simulink model "Simulator_3D"  (R2018a)
settings: Solver=ode4  StartTime=0.0  StopTime=80  FixedStep=T  RelTol=1e-3
values from neighbouring files (symbols this model uses):
  A_w = 1*1.5/2    (= 0.75)    [init_Simulator.m]
  A_w2 = 1*0.27/2    (= 0.135)    [init_Simulator.m]
  epsilon_w = 0    [init_Simulator.m]
  epsilon_w2 = pi    (= 3.14159265359)    [init_Simulator.m]
  k_w = omega_w^2/g    (= 0.123862835563)    [init_Simulator.m]
  k_w2 = omega_w2^2/g    (= 0.447144836384)    [init_Simulator.m]
  Lc_0 = 7    [init_Simulator.m]
  omega_w = 2*pi/T_w    (= 1.10231321179)    [init_Simulator.m]
  omega_w2 = 2*pi/T_w2    (= 2.09439510239)    [init_Simulator.m]
  T = 1/30    (= 0.0333333333333)    [init_Simulator.m]
  w_dir = 1    [init_Simulator.m]
  w_dir2 = 1    [init_Simulator.m]
  zu_bar = X0_b(2) + Lc_0*sin(alpha_bar_0)    [init_Simulator.m]
libraries: vrlib x132
(part 3 of 6)

== system Simulator_3D/Subsystem/5 static wave points6/Subsystem16 ==
  t : Inport
  x : Inport  Port=2
  Subsystem : Subsystem
  Subsystem1 : Subsystem
  Sum1 : Sum  Inputs=++|
  Sum2 : Sum  Inputs=++|
  zeta : Outport
  theta : Outport  Port=2
  wires:
  x/1 -> Subsystem/2(x), Subsystem1/2(x)
  t/1 -> Subsystem/1(t), Subsystem1/1(t)
  Subsystem/1(zeta(x,t)) -> Sum2/2
  Sum2/1 -> zeta/1
  Subsystem1/1(zeta(x,t)) -> Sum2/1
  Subsystem/2(theta) -> Sum1/2
  Subsystem1/2(theta) -> Sum1/1
  Sum1/1 -> theta/1

== system Simulator_3D/Subsystem/5 static wave points7/Subsystem12 ==
  t : Inport
  x : Inport  Port=2
  Subsystem : Subsystem
  Subsystem1 : Subsystem
  Sum1 : Sum  Inputs=++|
  Sum2 : Sum  Inputs=++|
  zeta : Outport
  theta : Outport  Port=2
  wires:
  x/1 -> Subsystem/2(x), Subsystem1/2(x)
  t/1 -> Subsystem/1(t), Subsystem1/1(t)
  Subsystem/1(zeta(x,t)) -> Sum2/2
  Sum2/1 -> zeta/1
  Subsystem1/1(zeta(x,t)) -> Sum2/1
  Subsystem/2(theta) -> Sum1/2
  Subsystem1/2(theta) -> Sum1/1
  Sum1/1 -> theta/1

== system Simulator_3D/Subsystem/5 static wave points7/Subsystem13 ==
  t : Inport
  x : Inport  Port=2
  Subsystem : Subsystem
  Subsystem1 : Subsystem
  Sum1 : Sum  Inputs=++|
  Sum2 : Sum  Inputs=++|
  zeta : Outport
  theta : Outport  Port=2
  wires:
  Sum1/1 -> theta/1
  Subsystem1/2(theta) -> Sum1/1
  Subsystem/2(theta) -> Sum1/2
  Subsystem1/1(zeta(x,t)) -> Sum2/1
  Sum2/1 -> zeta/1
  Subsystem/1(zeta(x,t)) -> Sum2/2
  t/1 -> Subsystem1/1(t), Subsystem/1(t)
  x/1 -> Subsystem1/2(x), Subsystem/2(x)

== system Simulator_3D/Subsystem/5 static wave points7/Subsystem14 ==
  t : Inport
  x : Inport  Port=2
  Subsystem : Subsystem
  Subsystem1 : Subsystem
  Sum1 : Sum  Inputs=++|
  Sum2 : Sum  Inputs=++|
  zeta : Outport
  theta : Outport  Port=2
  wires:
  x/1 -> Subsystem/2(x), Subsystem1/2(x)
  t/1 -> Subsystem/1(t), Subsystem1/1(t)
  Subsystem/1(zeta(x,t)) -> Sum2/2
  Sum2/1 -> zeta/1
  Subsystem1/1(zeta(x,t)) -> Sum2/1
  Subsystem/2(theta) -> Sum1/2
  Subsystem1/2(theta) -> Sum1/1
  Sum1/1 -> theta/1

== system Simulator_3D/Subsystem/5 static wave points7/Subsystem15 ==
  t : Inport
  x : Inport  Port=2
  Subsystem : Subsystem
  Subsystem1 : Subsystem
  Sum1 : Sum  Inputs=++|
  Sum2 : Sum  Inputs=++|
  zeta : Outport
  theta : Outport  Port=2
  wires:
  Sum1/1 -> theta/1
  Subsystem1/2(theta) -> Sum1/1
  Subsystem/2(theta) -> Sum1/2
  Subsystem1/1(zeta(x,t)) -> Sum2/1
  Sum2/1 -> zeta/1
  Subsystem/1(zeta(x,t)) -> Sum2/2
  t/1 -> Subsystem1/1(t), Subsystem/1(t)
  x/1 -> Subsystem1/2(x), Subsystem/2(x)

== system Simulator_3D/Subsystem/5 static wave points7/Subsystem16 ==
  t : Inport
  x : Inport  Port=2
  Subsystem : Subsystem
  Subsystem1 : Subsystem
  Sum1 : Sum  Inputs=++|
  Sum2 : Sum  Inputs=++|
  zeta : Outport
  theta : Outport  Port=2
  wires:
  x/1 -> Subsystem/2(x), Subsystem1/2(x)
  t/1 -> Subsystem/1(t), Subsystem1/1(t)
  Subsystem/1(zeta(x,t)) -> Sum2/2
  Sum2/1 -> zeta/1
  Subsystem1/1(zeta(x,t)) -> Sum2/1
  Subsystem/2(theta) -> Sum1/2
  Subsystem1/2(theta) -> Sum1/1
  Sum1/1 -> theta/1

== system Simulator_3D/Subsystem/5 static wave points7/crest1 ==
  t : Inport
  Constant : Constant  Value=epsilon_w
  Constant1 : Constant
  Constant2 : Constant  Value=-k_w
  Divide : Product  Inputs=*/
  Gain : Gain  Gain=omega_w
  Sum1 : Sum  Inputs=-+-
  Trigonometric Function2 : Trigonometry  Operator=asin
  direction : Gain  Gain=w_dir
  x crest : Outport
  wires:
  Gain/1 -> Sum1/1
  Constant/1 -> Sum1/3
  t/1 -> direction/1
  Constant2/1 -> Divide/2
  direction/1 -> Gain/1
  Constant1/1 -> Trigonometric Function2/1
  Trigonometric Function2/1 -> Sum1/2
  Sum1/1 -> Divide/1
  Divide/1 -> x crest/1

== system Simulator_3D/Subsystem/5 static wave points7/crest2 ==
  t : Inport
  Constant : Constant  Value=epsilon_w2
  Constant1 : Constant
  Constant2 : Constant  Value=-k_w2
  Divide : Product  Inputs=*/
  Gain : Gain  Gain=omega_w2
  Sum1 : Sum  Inputs=-+-
  Trigonometric Function2 : Trigonometry  Operator=asin
  direction : Gain  Gain=w_dir2
  x crest : Outport
  wires:
  Divide/1 -> x crest/1
  Sum1/1 -> Divide/1
  Trigonometric Function2/1 -> Sum1/2
  Constant1/1 -> Trigonometric Function2/1
  direction/1 -> Gain/1
  Constant2/1 -> Divide/2
  t/1 -> direction/1
  Constant/1 -> Sum1/3
  Gain/1 -> Sum1/1

== system Simulator_3D/Subsystem/followers/Subsystem1 ==
  t : Inport
  x : Inport  Port=2
  Subsystem : Subsystem
  Subsystem1 : Subsystem
  Sum1 : Sum  Inputs=++|
  Sum2 : Sum  Inputs=++|
  zeta : Outport
  theta : Outport  Port=2
  wires:
  Sum1/1 -> theta/1
  Subsystem1/2(theta) -> Sum1/1
  Subsystem/2(theta) -> Sum1/2
  Subsystem1/1(zeta(x,t)) -> Sum2/1
  Sum2/1 -> zeta/1
  Subsystem/1(zeta(x,t)) -> Sum2/2
  t/1 -> Subsystem1/1(t), Subsystem/1(t)
  x/1 -> Subsystem1/2(x), Subsystem/2(x)

== system Simulator_3D/Subsystem/followers/Subsystem2 ==
  t : Inport
  x : Inport  Port=2
  Subsystem : Subsystem
  Subsystem1 : Subsystem
  Sum1 : Sum  Inputs=++|
  Sum2 : Sum  Inputs=++|
  zeta : Outport
  theta : Outport  Port=2
  wires:
  x/1 -> Subsystem/2(x), Subsystem1/2(x)
  t/1 -> Subsystem/1(t), Subsystem1/1(t)
  Subsystem/1(zeta(x,t)) -> Sum2/2
  Sum2/1 -> zeta/1
  Subsystem1/1(zeta(x,t)) -> Sum2/1
  Subsystem/2(theta) -> Sum1/2
  Subsystem1/2(theta) -> Sum1/1
  Sum1/1 -> theta/1

== system Simulator_3D/Subsystem/followers/Subsystem3 ==
  t : Inport
  x : Inport  Port=2
  Subsystem : Subsystem
  Subsystem1 : Subsystem
  Sum1 : Sum  Inputs=++|
  Sum2 : Sum  Inputs=++|
  zeta : Outport
  theta : Outport  Port=2
  wires:
  x/1 -> Subsystem/2(x), Subsystem1/2(x)
  t/1 -> Subsystem/1(t), Subsystem1/1(t)
  Subsystem/1(zeta(x,t)) -> Sum2/2
  Sum2/1 -> zeta/1
  Subsystem1/1(zeta(x,t)) -> Sum2/1
  Subsystem/2(theta) -> Sum1/2
  Subsystem1/2(theta) -> Sum1/1
  Sum1/1 -> theta/1

== system Simulator_3D/Subsystem/followers/Subsystem4 ==
  t : Inport
  x : Inport  Port=2
  Subsystem : Subsystem
  Subsystem1 : Subsystem
  Sum1 : Sum  Inputs=++|
  Sum2 : Sum  Inputs=++|
  zeta : Outport
  theta : Outport  Port=2
  wires:
  Sum1/1 -> theta/1
  Subsystem1/2(theta) -> Sum1/1
  Subsystem/2(theta) -> Sum1/2
  Subsystem1/1(zeta(x,t)) -> Sum2/1
  Sum2/1 -> zeta/1
  Subsystem/1(zeta(x,t)) -> Sum2/2
  t/1 -> Subsystem1/1(t), Subsystem/1(t)
  x/1 -> Subsystem1/2(x), Subsystem/2(x)

== system Simulator_3D/Subsystem/followers/Subsystem5 ==
  t : Inport
  x : Inport  Port=2
  Subsystem : Subsystem
  Subsystem1 : Subsystem
  Sum1 : Sum  Inputs=++|
  Sum2 : Sum  Inputs=++|
  zeta : Outport
  theta : Outport  Port=2
  wires:
  x/1 -> Subsystem/2(x), Subsystem1/2(x)
  t/1 -> Subsystem/1(t), Subsystem1/1(t)
  Subsystem/1(zeta(x,t)) -> Sum2/2
  Sum2/1 -> zeta/1
  Subsystem1/1(zeta(x,t)) -> Sum2/1
  Subsystem/2(theta) -> Sum1/2
  Subsystem1/2(theta) -> Sum1/1
  Sum1/1 -> theta/1

== system Simulator_3D/Subsystem/followers/Subsystem6 ==
  t : Inport
  x : Inport  Port=2
  Subsystem : Subsystem
  Subsystem1 : Subsystem
  Sum1 : Sum  Inputs=++|
  Sum2 : Sum  Inputs=++|
  zeta : Outport
  theta : Outport  Port=2
  wires:
  Sum1/1 -> theta/1
  Subsystem1/2(theta) -> Sum1/1
  Subsystem/2(theta) -> Sum1/2
  Subsystem1/1(zeta(x,t)) -> Sum2/1
  Sum2/1 -> zeta/1
  Subsystem/1(zeta(x,t)) -> Sum2/2
  t/1 -> Subsystem1/1(t), Subsystem/1(t)
  x/1 -> Subsystem1/2(x), Subsystem/2(x)

== system Simulator_3D/Subsystem/followers/Subsystem7 ==
  t : Inport
  x : Inport  Port=2
  Subsystem : Subsystem
  Subsystem1 : Subsystem
  Sum1 : Sum  Inputs=++|
  Sum2 : Sum  Inputs=++|
  zeta : Outport
  theta : Outport  Port=2
  wires:
  x/1 -> Subsystem/2(x), Subsystem1/2(x)
  t/1 -> Subsystem/1(t), Subsystem1/1(t)
  Subsystem/1(zeta(x,t)) -> Sum2/2
  Sum2/1 -> zeta/1
  Subsystem1/1(zeta(x,t)) -> Sum2/1
  Subsystem/2(theta) -> Sum1/2
  Subsystem1/2(theta) -> Sum1/1
  Sum1/1 -> theta/1

== system Simulator_3D/Subsystem/followers/Subsystem8 ==
  t : Inport
  x : Inport  Port=2
  Subsystem : Subsystem
  Subsystem1 : Subsystem
  Sum1 : Sum  Inputs=++|
  Sum2 : Sum  Inputs=++|
  zeta : Outport
  theta : Outport  Port=2
  wires:
  Sum1/1 -> theta/1
  Subsystem1/2(theta) -> Sum1/1
  Subsystem/2(theta) -> Sum1/2
  Subsystem1/1(zeta(x,t)) -> Sum2/1
  Sum2/1 -> zeta/1
  Subsystem/1(zeta(x,t)) -> Sum2/2
  t/1 -> Subsystem1/1(t), Subsystem/1(t)
  x/1 -> Subsystem1/2(x), Subsystem/2(x)

== system Simulator_3D/Subsystem1/Subsystem1/Subsystem ==
  note: Aw.Sin
  t : Inport
  x : Inport  Port=2
  Constant : Constant  Value=epsilon_w
  Gain : Gain  Gain=omega_w
  Gain1 : Gain  Gain=k_w
  Gain2 : Gain  Gain=A_w
  Sum : Sum  Inputs=++-
  Trigonometric Function : Trigonometry
  direction : Gain  Gain=w_dir
  zeta(x,t) : Outport
  wires:
  Gain/1 -> Sum/2
  Gain2/1 -> zeta(x,t)/1  "zeta(x,t)"
  Constant/1 -> Sum/1
  t/1 -> direction/1
  Gain1/1 -> Sum/3
  Trigonometric Function/1 -> Gain2/1
  x/1 -> Gain1/1
  direction/1 -> Gain/1
  Sum/1 -> Trigonometric Function/1

== system Simulator_3D/Subsystem1/Subsystem1/Subsystem1 ==
  note: Aw.Sin
  t : Inport
  x : Inport  Port=2
  Constant : Constant  Value=epsilon_w2
  Gain : Gain  Gain=omega_w2
  Gain1 : Gain  Gain=k_w2
  Gain2 : Gain  Gain=A_w2
  Sum : Sum  Inputs=++-
  Trigonometric Function : Trigonometry
  direction : Gain  Gain=w_dir2
  zeta(x,t) : Outport
  wires:
  Sum/1 -> Trigonometric Function/1
  direction/1 -> Gain/1
  x/1 -> Gain1/1
  Trigonometric Function/1 -> Gain2/1
  Gain1/1 -> Sum/3
  t/1 -> direction/1
  Constant/1 -> Sum/1
  Gain2/1 -> zeta(x,t)/1  "zeta(x,t)"
  Gain/1 -> Sum/2

== system Simulator_3D/Subsystem1/Subsystem10/Subsystem ==
  note: Aw.Sin
  t : Inport
  x : Inport  Port=2
  Constant : Constant  Value=epsilon_w
  Gain : Gain  Gain=omega_w
  Gain1 : Gain  Gain=k_w
  Gain2 : Gain  Gain=A_w
  Sum : Sum  Inputs=++-
  Trigonometric Function : Trigonometry
  direction : Gain  Gain=w_dir
  zeta(x,t) : Outport
  wires:
  Sum/1 -> Trigonometric Function/1
  direction/1 -> Gain/1
  x/1 -> Gain1/1
  Trigonometric Function/1 -> Gain2/1
  Gain1/1 -> Sum/3
  t/1 -> direction/1
  Constant/1 -> Sum/1
  Gain2/1 -> zeta(x,t)/1  "zeta(x,t)"
  Gain/1 -> Sum/2

== system Simulator_3D/Subsystem1/Subsystem10/Subsystem1 ==
  note: Aw.Sin
  t : Inport
  x : Inport  Port=2
  Constant : Constant  Value=epsilon_w2
  Gain : Gain  Gain=omega_w2
  Gain1 : Gain  Gain=k_w2
  Gain2 : Gain  Gain=A_w2
  Sum : Sum  Inputs=++-
  Trigonometric Function : Trigonometry
  direction : Gain  Gain=w_dir2
  zeta(x,t) : Outport
  wires:
  Gain/1 -> Sum/2
  Gain2/1 -> zeta(x,t)/1  "zeta(x,t)"
  Constant/1 -> Sum/1
  t/1 -> direction/1
  Gain1/1 -> Sum/3
  Trigonometric Function/1 -> Gain2/1
  x/1 -> Gain1/1
  direction/1 -> Gain/1
  Sum/1 -> Trigonometric Function/1

== system Simulator_3D/Subsystem1/Subsystem11/Subsystem ==
  note: Aw.Sin
  t : Inport
  x : Inport  Port=2
  Constant : Constant  Value=epsilon_w
  Gain : Gain  Gain=omega_w
  Gain1 : Gain  Gain=k_w
  Gain2 : Gain  Gain=A_w
  Sum : Sum  Inputs=++-
  Trigonometric Function : Trigonometry
  direction : Gain  Gain=w_dir
  zeta(x,t) : Outport
  wires:
  Gain/1 -> Sum/2
  Gain2/1 -> zeta(x,t)/1  "zeta(x,t)"
  Constant/1 -> Sum/1
  t/1 -> direction/1
  Gain1/1 -> Sum/3
  Trigonometric Function/1 -> Gain2/1
  x/1 -> Gain1/1
  direction/1 -> Gain/1
  Sum/1 -> Trigonometric Function/1

== system Simulator_3D/Subsystem1/Subsystem11/Subsystem1 ==
  note: Aw.Sin
  t : Inport
  x : Inport  Port=2
  Constant : Constant  Value=epsilon_w2
  Gain : Gain  Gain=omega_w2
  Gain1 : Gain  Gain=k_w2
  Gain2 : Gain  Gain=A_w2
  Sum : Sum  Inputs=++-
  Trigonometric Function : Trigonometry
  direction : Gain  Gain=w_dir2
  zeta(x,t) : Outport
  wires:
  Sum/1 -> Trigonometric Function/1
  direction/1 -> Gain/1
  x/1 -> Gain1/1
  Trigonometric Function/1 -> Gain2/1
  Gain1/1 -> Sum/3
  t/1 -> direction/1
  Constant/1 -> Sum/1
  Gain2/1 -> zeta(x,t)/1  "zeta(x,t)"
  Gain/1 -> Sum/2

== system Simulator_3D/Subsystem1/Subsystem12/Subsystem ==
  note: Aw.Sin
  t : Inport
  x : Inport  Port=2
  Constant : Constant  Value=epsilon_w
  Gain : Gain  Gain=omega_w
  Gain1 : Gain  Gain=k_w
  Gain2 : Gain  Gain=A_w
  Sum : Sum  Inputs=++-
  Trigonometric Function : Trigonometry
  direction : Gain  Gain=w_dir
  zeta(x,t) : Outport
  wires:
  Sum/1 -> Trigonometric Function/1
  direction/1 -> Gain/1
  x/1 -> Gain1/1
  Trigonometric Function/1 -> Gain2/1
  Gain1/1 -> Sum/3
  t/1 -> direction/1
  Constant/1 -> Sum/1
  Gain2/1 -> zeta(x,t)/1  "zeta(x,t)"
  Gain/1 -> Sum/2

== system Simulator_3D/Subsystem1/Subsystem12/Subsystem1 ==
  note: Aw.Sin
  t : Inport
  x : Inport  Port=2
  Constant : Constant  Value=epsilon_w2
  Gain : Gain  Gain=omega_w2
  Gain1 : Gain  Gain=k_w2
  Gain2 : Gain  Gain=A_w2
  Sum : Sum  Inputs=++-
  Trigonometric Function : Trigonometry
  direction : Gain  Gain=w_dir2
  zeta(x,t) : Outport
  wires:
  Gain/1 -> Sum/2
  Gain2/1 -> zeta(x,t)/1  "zeta(x,t)"
  Constant/1 -> Sum/1
  t/1 -> direction/1
  Gain1/1 -> Sum/3
  Trigonometric Function/1 -> Gain2/1
  x/1 -> Gain1/1
  direction/1 -> Gain/1
  Sum/1 -> Trigonometric Function/1

== system Simulator_3D/Subsystem1/Subsystem13/Subsystem ==
  note: Aw.Sin
  t : Inport
  x : Inport  Port=2
  Constant : Constant  Value=epsilon_w
  Gain : Gain  Gain=omega_w
  Gain1 : Gain  Gain=k_w
  Gain2 : Gain  Gain=A_w
  Sum : Sum  Inputs=++-
  Trigonometric Function : Trigonometry
  direction : Gain  Gain=w_dir
  zeta(x,t) : Outport
  wires:
  Gain/1 -> Sum/2
  Gain2/1 -> zeta(x,t)/1  "zeta(x,t)"
  Constant/1 -> Sum/1
  t/1 -> direction/1
  Gain1/1 -> Sum/3
  Trigonometric Function/1 -> Gain2/1
  x/1 -> Gain1/1
  direction/1 -> Gain/1
  Sum/1 -> Trigonometric Function/1

== system Simulator_3D/Subsystem1/Subsystem13/Subsystem1 ==
  note: Aw.Sin
  t : Inport
  x : Inport  Port=2
  Constant : Constant  Value=epsilon_w2
  Gain : Gain  Gain=omega_w2
  Gain1 : Gain  Gain=k_w2
  Gain2 : Gain  Gain=A_w2
  Sum : Sum  Inputs=++-
  Trigonometric Function : Trigonometry
  direction : Gain  Gain=w_dir2
  zeta(x,t) : Outport
  wires:
  Sum/1 -> Trigonometric Function/1
  direction/1 -> Gain/1
  x/1 -> Gain1/1
  Trigonometric Function/1 -> Gain2/1
  Gain1/1 -> Sum/3
  t/1 -> direction/1
  Constant/1 -> Sum/1
  Gain2/1 -> zeta(x,t)/1  "zeta(x,t)"
  Gain/1 -> Sum/2

== system Simulator_3D/Subsystem1/Subsystem14/Subsystem ==
  note: Aw.Sin
  t : Inport
  x : Inport  Port=2
  Constant : Constant  Value=epsilon_w
  Gain : Gain  Gain=omega_w
  Gain1 : Gain  Gain=k_w
  Gain2 : Gain  Gain=A_w
  Sum : Sum  Inputs=++-
  Trigonometric Function : Trigonometry
  direction : Gain  Gain=w_dir
  zeta(x,t) : Outport
  wires:
  Sum/1 -> Trigonometric Function/1
  direction/1 -> Gain/1
  x/1 -> Gain1/1
  Trigonometric Function/1 -> Gain2/1
  Gain1/1 -> Sum/3
  t/1 -> direction/1
  Constant/1 -> Sum/1
  Gain2/1 -> zeta(x,t)/1  "zeta(x,t)"
  Gain/1 -> Sum/2

== system Simulator_3D/Subsystem1/Subsystem14/Subsystem1 ==
  note: Aw.Sin
  t : Inport
  x : Inport  Port=2
  Constant : Constant  Value=epsilon_w2
  Gain : Gain  Gain=omega_w2
  Gain1 : Gain  Gain=k_w2
  Gain2 : Gain  Gain=A_w2
  Sum : Sum  Inputs=++-
  Trigonometric Function : Trigonometry
  direction : Gain  Gain=w_dir2
  zeta(x,t) : Outport
  wires:
  Gain/1 -> Sum/2
  Gain2/1 -> zeta(x,t)/1  "zeta(x,t)"
  Constant/1 -> Sum/1
  t/1 -> direction/1
  Gain1/1 -> Sum/3
  Trigonometric Function/1 -> Gain2/1
  x/1 -> Gain1/1
  direction/1 -> Gain/1
  Sum/1 -> Trigonometric Function/1

== system Simulator_3D/Subsystem1/Subsystem15/Subsystem ==
  note: Aw.Sin
  t : Inport
  x : Inport  Port=2
  Constant : Constant  Value=epsilon_w
  Gain : Gain  Gain=omega_w
  Gain1 : Gain  Gain=k_w
  Gain2 : Gain  Gain=A_w
  Sum : Sum  Inputs=++-
  Trigonometric Function : Trigonometry
  direction : Gain  Gain=w_dir
  zeta(x,t) : Outport
  wires:
  Gain/1 -> Sum/2
  Gain2/1 -> zeta(x,t)/1  "zeta(x,t)"
  Constant/1 -> Sum/1
  t/1 -> direction/1
  Gain1/1 -> Sum/3
  Trigonometric Function/1 -> Gain2/1
  x/1 -> Gain1/1
  direction/1 -> Gain/1
  Sum/1 -> Trigonometric Function/1

== system Simulator_3D/Subsystem1/Subsystem15/Subsystem1 ==
  note: Aw.Sin
  t : Inport
  x : Inport  Port=2
  Constant : Constant  Value=epsilon_w2
  Gain : Gain  Gain=omega_w2
  Gain1 : Gain  Gain=k_w2
  Gain2 : Gain  Gain=A_w2
  Sum : Sum  Inputs=++-
  Trigonometric Function : Trigonometry
  direction : Gain  Gain=w_dir2
  zeta(x,t) : Outport
  wires:
  Sum/1 -> Trigonometric Function/1
  direction/1 -> Gain/1
  x/1 -> Gain1/1
  Trigonometric Function/1 -> Gain2/1
  Gain1/1 -> Sum/3
  t/1 -> direction/1
  Constant/1 -> Sum/1
  Gain2/1 -> zeta(x,t)/1  "zeta(x,t)"
  Gain/1 -> Sum/2

== system Simulator_3D/Subsystem1/Subsystem16/Subsystem ==
  note: Aw.Sin
  t : Inport
  x : Inport  Port=2
  Constant : Constant  Value=epsilon_w
  Gain : Gain  Gain=omega_w
  Gain1 : Gain  Gain=k_w
  Gain2 : Gain  Gain=A_w
  Sum : Sum  Inputs=++-
  Trigonometric Function : Trigonometry
  direction : Gain  Gain=w_dir
  zeta(x,t) : Outport
  wires:
  Sum/1 -> Trigonometric Function/1
  direction/1 -> Gain/1
  x/1 -> Gain1/1
  Trigonometric Function/1 -> Gain2/1
  Gain1/1 -> Sum/3
  t/1 -> direction/1
  Constant/1 -> Sum/1
  Gain2/1 -> zeta(x,t)/1  "zeta(x,t)"
  Gain/1 -> Sum/2

== system Simulator_3D/Subsystem1/Subsystem16/Subsystem1 ==
  note: Aw.Sin
  t : Inport
  x : Inport  Port=2
  Constant : Constant  Value=epsilon_w2
  Gain : Gain  Gain=omega_w2
  Gain1 : Gain  Gain=k_w2
  Gain2 : Gain  Gain=A_w2
  Sum : Sum  Inputs=++-
  Trigonometric Function : Trigonometry
  direction : Gain  Gain=w_dir2
  zeta(x,t) : Outport
  wires:
  Gain/1 -> Sum/2
  Gain2/1 -> zeta(x,t)/1  "zeta(x,t)"
  Constant/1 -> Sum/1
  t/1 -> direction/1
  Gain1/1 -> Sum/3
  Trigonometric Function/1 -> Gain2/1
  x/1 -> Gain1/1
  direction/1 -> Gain/1
  Sum/1 -> Trigonometric Function/1

== system Simulator_3D/Subsystem1/Subsystem2/Subsystem ==
  note: Aw.Sin
  t : Inport
  x : Inport  Port=2
  Constant : Constant  Value=epsilon_w
  Gain : Gain  Gain=omega_w
  Gain1 : Gain  Gain=k_w
  Gain2 : Gain  Gain=A_w
  Sum : Sum  Inputs=++-
  Trigonometric Function : Trigonometry
  direction : Gain  Gain=w_dir
  zeta(x,t) : Outport
  wires:
  Sum/1 -> Trigonometric Function/1
  direction/1 -> Gain/1
  x/1 -> Gain1/1
  Trigonometric Function/1 -> Gain2/1
  Gain1/1 -> Sum/3
  t/1 -> direction/1
  Constant/1 -> Sum/1
  Gain2/1 -> zeta(x,t)/1  "zeta(x,t)"
  Gain/1 -> Sum/2

== system Simulator_3D/Subsystem1/Subsystem2/Subsystem1 ==
  note: Aw.Sin
  t : Inport
  x : Inport  Port=2
  Constant : Constant  Value=epsilon_w2
  Gain : Gain  Gain=omega_w2
  Gain1 : Gain  Gain=k_w2
  Gain2 : Gain  Gain=A_w2
  Sum : Sum  Inputs=++-
  Trigonometric Function : Trigonometry
  direction : Gain  Gain=w_dir2
  zeta(x,t) : Outport
  wires:
  Gain/1 -> Sum/2
  Gain2/1 -> zeta(x,t)/1  "zeta(x,t)"
  Constant/1 -> Sum/1
  t/1 -> direction/1
  Gain1/1 -> Sum/3
  Trigonometric Function/1 -> Gain2/1
  x/1 -> Gain1/1
  direction/1 -> Gain/1
  Sum/1 -> Trigonometric Function/1

== system Simulator_3D/Subsystem1/Subsystem3/Subsystem ==
  note: Aw.Sin
  t : Inport
  x : Inport  Port=2
  Constant : Constant  Value=epsilon_w
  Gain : Gain  Gain=omega_w
  Gain1 : Gain  Gain=k_w
  Gain2 : Gain  Gain=A_w
  Sum : Sum  Inputs=++-
  Trigonometric Function : Trigonometry
  direction : Gain  Gain=w_dir
  zeta(x,t) : Outport
  wires:
  Gain/1 -> Sum/2
  Gain2/1 -> zeta(x,t)/1  "zeta(x,t)"
  Constant/1 -> Sum/1
  t/1 -> direction/1
  Gain1/1 -> Sum/3
  Trigonometric Function/1 -> Gain2/1
  x/1 -> Gain1/1
  direction/1 -> Gain/1
  Sum/1 -> Trigonometric Function/1

== system Simulator_3D/Subsystem1/Subsystem3/Subsystem1 ==
  note: Aw.Sin
  t : Inport
  x : Inport  Port=2
  Constant : Constant  Value=epsilon_w2
  Gain : Gain  Gain=omega_w2
  Gain1 : Gain  Gain=k_w2
  Gain2 : Gain  Gain=A_w2
  Sum : Sum  Inputs=++-
  Trigonometric Function : Trigonometry
  direction : Gain  Gain=w_dir2
  zeta(x,t) : Outport
  wires:
  Sum/1 -> Trigonometric Function/1
  direction/1 -> Gain/1
  x/1 -> Gain1/1
  Trigonometric Function/1 -> Gain2/1
  Gain1/1 -> Sum/3
  t/1 -> direction/1
  Constant/1 -> Sum/1
  Gain2/1 -> zeta(x,t)/1  "zeta(x,t)"
  Gain/1 -> Sum/2

== system Simulator_3D/Subsystem1/Subsystem4/Subsystem ==
  note: Aw.Sin
  t : Inport
  x : Inport  Port=2
  Constant : Constant  Value=epsilon_w
  Gain : Gain  Gain=omega_w
  Gain1 : Gain  Gain=k_w
  Gain2 : Gain  Gain=A_w
  Sum : Sum  Inputs=++-
  Trigonometric Function : Trigonometry
  direction : Gain  Gain=w_dir
  zeta(x,t) : Outport
  wires:
  Sum/1 -> Trigonometric Function/1
  direction/1 -> Gain/1
  x/1 -> Gain1/1
  Trigonometric Function/1 -> Gain2/1
  Gain1/1 -> Sum/3
  t/1 -> direction/1
  Constant/1 -> Sum/1
  Gain2/1 -> zeta(x,t)/1  "zeta(x,t)"
  Gain/1 -> Sum/2

== system Simulator_3D/Subsystem1/Subsystem4/Subsystem1 ==
  note: Aw.Sin
  t : Inport
  x : Inport  Port=2
  Constant : Constant  Value=epsilon_w2
  Gain : Gain  Gain=omega_w2
  Gain1 : Gain  Gain=k_w2
  Gain2 : Gain  Gain=A_w2
  Sum : Sum  Inputs=++-
  Trigonometric Function : Trigonometry
  direction : Gain  Gain=w_dir2
  zeta(x,t) : Outport
  wires:
  Gain/1 -> Sum/2
  Gain2/1 -> zeta(x,t)/1  "zeta(x,t)"
  Constant/1 -> Sum/1
  t/1 -> direction/1
  Gain1/1 -> Sum/3
  Trigonometric Function/1 -> Gain2/1
  x/1 -> Gain1/1
  direction/1 -> Gain/1
  Sum/1 -> Trigonometric Function/1

== system Simulator_3D/Subsystem1/Subsystem5/Subsystem ==
  note: Aw.Sin
  t : Inport
  x : Inport  Port=2
  Constant : Constant  Value=epsilon_w
  Gain : Gain  Gain=omega_w
  Gain1 : Gain  Gain=k_w
  Gain2 : Gain  Gain=A_w
  Sum : Sum  Inputs=++-
  Trigonometric Function : Trigonometry
  direction : Gain  Gain=w_dir
  zeta(x,t) : Outport
  wires:
  Gain/1 -> Sum/2
  Gain2/1 -> zeta(x,t)/1  "zeta(x,t)"
  Constant/1 -> Sum/1
  t/1 -> direction/1
  Gain1/1 -> Sum/3
  Trigonometric Function/1 -> Gain2/1
  x/1 -> Gain1/1
  direction/1 -> Gain/1
  Sum/1 -> Trigonometric Function/1

== system Simulator_3D/Subsystem1/Subsystem5/Subsystem1 ==
  note: Aw.Sin
  t : Inport
  x : Inport  Port=2
  Constant : Constant  Value=epsilon_w2
  Gain : Gain  Gain=omega_w2
  Gain1 : Gain  Gain=k_w2
  Gain2 : Gain  Gain=A_w2
  Sum : Sum  Inputs=++-
  Trigonometric Function : Trigonometry
  direction : Gain  Gain=w_dir2
  zeta(x,t) : Outport
  wires:
  Sum/1 -> Trigonometric Function/1
  direction/1 -> Gain/1
  x/1 -> Gain1/1
  Trigonometric Function/1 -> Gain2/1
  Gain1/1 -> Sum/3
  t/1 -> direction/1
  Constant/1 -> Sum/1
  Gain2/1 -> zeta(x,t)/1  "zeta(x,t)"
  Gain/1 -> Sum/2

== system Simulator_3D/Subsystem1/Subsystem6/Subsystem ==
  note: Aw.Sin
  t : Inport
  x : Inport  Port=2
  Constant : Constant  Value=epsilon_w
  Gain : Gain  Gain=omega_w
  Gain1 : Gain  Gain=k_w
  Gain2 : Gain  Gain=A_w
  Sum : Sum  Inputs=++-
  Trigonometric Function : Trigonometry
  direction : Gain  Gain=w_dir
  zeta(x,t) : Outport
  wires:
  Sum/1 -> Trigonometric Function/1
  direction/1 -> Gain/1
  x/1 -> Gain1/1
  Trigonometric Function/1 -> Gain2/1
  Gain1/1 -> Sum/3
  t/1 -> direction/1
  Constant/1 -> Sum/1
  Gain2/1 -> zeta(x,t)/1  "zeta(x,t)"
  Gain/1 -> Sum/2

== system Simulator_3D/Subsystem1/Subsystem6/Subsystem1 ==
  note: Aw.Sin
  t : Inport
  x : Inport  Port=2
  Constant : Constant  Value=epsilon_w2
  Gain : Gain  Gain=omega_w2
  Gain1 : Gain  Gain=k_w2
  Gain2 : Gain  Gain=A_w2
  Sum : Sum  Inputs=++-
  Trigonometric Function : Trigonometry
  direction : Gain  Gain=w_dir2
  zeta(x,t) : Outport
  wires:
  Gain/1 -> Sum/2
  Gain2/1 -> zeta(x,t)/1  "zeta(x,t)"
  Constant/1 -> Sum/1
  t/1 -> direction/1
  Gain1/1 -> Sum/3
  Trigonometric Function/1 -> Gain2/1
  x/1 -> Gain1/1
  direction/1 -> Gain/1
  Sum/1 -> Trigonometric Function/1

== system Simulator_3D/Subsystem1/Subsystem7/Subsystem ==
  note: Aw.Sin
  t : Inport
  x : Inport  Port=2
  Constant : Constant  Value=epsilon_w
  Gain : Gain  Gain=omega_w
  Gain1 : Gain  Gain=k_w
  Gain2 : Gain  Gain=A_w
  Sum : Sum  Inputs=++-
  Trigonometric Function : Trigonometry
  direction : Gain  Gain=w_dir
  zeta(x,t) : Outport
  wires:
  Gain/1 -> Sum/2
  Gain2/1 -> zeta(x,t)/1  "zeta(x,t)"
  Constant/1 -> Sum/1
  t/1 -> direction/1
  Gain1/1 -> Sum/3
  Trigonometric Function/1 -> Gain2/1
  x/1 -> Gain1/1
  direction/1 -> Gain/1
  Sum/1 -> Trigonometric Function/1

== system Simulator_3D/Subsystem1/Subsystem7/Subsystem1 ==
  note: Aw.Sin
  t : Inport
  x : Inport  Port=2
  Constant : Constant  Value=epsilon_w2
  Gain : Gain  Gain=omega_w2
  Gain1 : Gain  Gain=k_w2
  Gain2 : Gain  Gain=A_w2
  Sum : Sum  Inputs=++-
  Trigonometric Function : Trigonometry
  direction : Gain  Gain=w_dir2
  zeta(x,t) : Outport
  wires:
  Sum/1 -> Trigonometric Function/1
  direction/1 -> Gain/1
  x/1 -> Gain1/1
  Trigonometric Function/1 -> Gain2/1
  Gain1/1 -> Sum/3
  t/1 -> direction/1
  Constant/1 -> Sum/1
  Gain2/1 -> zeta(x,t)/1  "zeta(x,t)"
  Gain/1 -> Sum/2

== system Simulator_3D/Subsystem1/Subsystem8/Subsystem ==
  note: Aw.Sin
  t : Inport
  x : Inport  Port=2
  Constant : Constant  Value=epsilon_w
  Gain : Gain  Gain=omega_w
  Gain1 : Gain  Gain=k_w
  Gain2 : Gain  Gain=A_w
  Sum : Sum  Inputs=++-
  Trigonometric Function : Trigonometry
  direction : Gain  Gain=w_dir
  zeta(x,t) : Outport
  wires:
  Sum/1 -> Trigonometric Function/1
  direction/1 -> Gain/1
  x/1 -> Gain1/1
  Trigonometric Function/1 -> Gain2/1
  Gain1/1 -> Sum/3
  t/1 -> direction/1
  Constant/1 -> Sum/1
  Gain2/1 -> zeta(x,t)/1  "zeta(x,t)"
  Gain/1 -> Sum/2

== system Simulator_3D/Subsystem1/Subsystem8/Subsystem1 ==
  note: Aw.Sin
  t : Inport
  x : Inport  Port=2
  Constant : Constant  Value=epsilon_w2
  Gain : Gain  Gain=omega_w2
  Gain1 : Gain  Gain=k_w2
  Gain2 : Gain  Gain=A_w2
  Sum : Sum  Inputs=++-
  Trigonometric Function : Trigonometry
  direction : Gain  Gain=w_dir2
  zeta(x,t) : Outport
  wires:
  Gain/1 -> Sum/2
  Gain2/1 -> zeta(x,t)/1  "zeta(x,t)"
  Constant/1 -> Sum/1
  t/1 -> direction/1
  Gain1/1 -> Sum/3
  Trigonometric Function/1 -> Gain2/1
  x/1 -> Gain1/1
  direction/1 -> Gain/1
  Sum/1 -> Trigonometric Function/1

== system Simulator_3D/Subsystem1/Subsystem9/Subsystem ==
  note: Aw.Sin
  t : Inport
  x : Inport  Port=2
  Constant : Constant  Value=epsilon_w
  Gain : Gain  Gain=omega_w
  Gain1 : Gain  Gain=k_w
  Gain2 : Gain  Gain=A_w
  Sum : Sum  Inputs=++-
  Trigonometric Function : Trigonometry
  direction : Gain  Gain=w_dir
  zeta(x,t) : Outport
  wires:
  Gain/1 -> Sum/2
  Gain2/1 -> zeta(x,t)/1  "zeta(x,t)"
  Constant/1 -> Sum/1
  t/1 -> direction/1
  Gain1/1 -> Sum/3
  Trigonometric Function/1 -> Gain2/1
  x/1 -> Gain1/1
  direction/1 -> Gain/1
  Sum/1 -> Trigonometric Function/1

== system Simulator_3D/Subsystem1/Subsystem9/Subsystem1 ==
  note: Aw.Sin
  t : Inport
  x : Inport  Port=2
  Constant : Constant  Value=epsilon_w2
  Gain : Gain  Gain=omega_w2
  Gain1 : Gain  Gain=k_w2
  Gain2 : Gain  Gain=A_w2
  Sum : Sum  Inputs=++-
  Trigonometric Function : Trigonometry
  direction : Gain  Gain=w_dir2
  zeta(x,t) : Outport
  wires:
  Sum/1 -> Trigonometric Function/1
  direction/1 -> Gain/1
  x/1 -> Gain1/1
  Trigonometric Function/1 -> Gain2/1
  Gain1/1 -> Sum/3
  t/1 -> direction/1
  Constant/1 -> Sum/1
  Gain2/1 -> zeta(x,t)/1  "zeta(x,t)"
  Gain/1 -> Sum/2

== system Simulator_3D/Subsystem2/Subsystem1/Subsystem ==
  note: Aw.Sin
  t : Inport
  x : Inport  Port=2
  Constant : Constant  Value=epsilon_w
  Gain : Gain  Gain=omega_w
  Gain1 : Gain  Gain=k_w
  Gain2 : Gain  Gain=A_w
  Gain5 : Gain  Gain=A_w*k_w
  Sum : Sum  Inputs=++-
  Trigonometric Function1 : Trigonometry  Operator=sincos
  Trigonometric Function2 : Trigonometry  Operator=atan
  direction : Gain  Gain=w_dir
  zeta(x,t) : Outport
  theta : Outport  Port=2
  wires:
  Trigonometric Function2/1 -> theta/1
  Gain5/1 -> Trigonometric Function2/1
  Trigonometric Function1/2 -> Gain5/1
  Gain/1 -> Sum/2
  Gain2/1 -> zeta(x,t)/1  "zeta(x,t)"
  Constant/1 -> Sum/1
  t/1 -> direction/1
  Gain1/1 -> Sum/3
  Trigonometric Function1/1 -> Gain2/1
  x/1 -> Gain1/1
  direction/1 -> Gain/1
  Sum/1 -> Trigonometric Function1/1

== system Simulator_3D/Subsystem2/Subsystem1/Subsystem1 ==
  note: Aw.Sin
  t : Inport
  x : Inport  Port=2
  Constant : Constant  Value=epsilon_w2
  Gain : Gain  Gain=omega_w2
  Gain1 : Gain  Gain=k_w2
  Gain2 : Gain  Gain=A_w2
  Gain5 : Gain  Gain=A_w2*k_w2
  Sum : Sum  Inputs=++-
  Trigonometric Function : Trigonometry  Operator=sincos
  Trigonometric Function1 : Trigonometry  Operator=atan
  direction : Gain  Gain=w_dir2
  zeta(x,t) : Outport
  theta : Outport  Port=2
  wires:
  Trigonometric Function/2 -> Gain5/1
  Trigonometric Function1/1 -> theta/1
  Gain5/1 -> Trigonometric Function1/1
  Sum/1 -> Trigonometric Function/1
  direction/1 -> Gain/1
  x/1 -> Gain1/1
  Trigonometric Function/1 -> Gain2/1
  Gain1/1 -> Sum/3
  t/1 -> direction/1
  Constant/1 -> Sum/1
  Gain2/1 -> zeta(x,t)/1  "zeta(x,t)"
  Gain/1 -> Sum/2

== system Simulator_3D/Subsystem2/Subsystem10/Subsystem ==
  note: Aw.Sin
  t : Inport
  x : Inport  Port=2
  Constant : Constant  Value=epsilon_w
  Gain : Gain  Gain=omega_w
  Gain1 : Gain  Gain=k_w
  Gain2 : Gain  Gain=A_w
  Gain5 : Gain  Gain=A_w*k_w
  Sum : Sum  Inputs=++-
  Trigonometric Function1 : Trigonometry  Operator=sincos
  Trigonometric Function2 : Trigonometry  Operator=atan
  direction : Gain  Gain=w_dir
  zeta(x,t) : Outport
  theta : Outport  Port=2
  wires:
  Trigonometric Function2/1 -> theta/1
  Gain5/1 -> Trigonometric Function2/1
  Trigonometric Function1/2 -> Gain5/1
  Gain/1 -> Sum/2
  Gain2/1 -> zeta(x,t)/1  "zeta(x,t)"
  Constant/1 -> Sum/1
  t/1 -> direction/1
  Gain1/1 -> Sum/3
  Trigonometric Function1/1 -> Gain2/1
  x/1 -> Gain1/1
  direction/1 -> Gain/1
  Sum/1 -> Trigonometric Function1/1

== system Simulator_3D/Subsystem2/Subsystem10/Subsystem1 ==
  note: Aw.Sin
  t : Inport
  x : Inport  Port=2
  Constant : Constant  Value=epsilon_w2
  Gain : Gain  Gain=omega_w2
  Gain1 : Gain  Gain=k_w2
  Gain2 : Gain  Gain=A_w2
  Gain5 : Gain  Gain=A_w2*k_w2
  Sum : Sum  Inputs=++-
  Trigonometric Function : Trigonometry  Operator=sincos
  Trigonometric Function1 : Trigonometry  Operator=atan
  direction : Gain  Gain=w_dir2
  zeta(x,t) : Outport
  theta : Outport  Port=2
  wires:
  Trigonometric Function/2 -> Gain5/1
  Trigonometric Function1/1 -> theta/1
  Gain5/1 -> Trigonometric Function1/1
  Sum/1 -> Trigonometric Function/1
  direction/1 -> Gain/1
  x/1 -> Gain1/1
  Trigonometric Function/1 -> Gain2/1
  Gain1/1 -> Sum/3
  t/1 -> direction/1
  Constant/1 -> Sum/1
  Gain2/1 -> zeta(x,t)/1  "zeta(x,t)"
  Gain/1 -> Sum/2

== system Simulator_3D/Subsystem2/Subsystem11/Subsystem ==
  note: Aw.Sin
  t : Inport
  x : Inport  Port=2
  Constant : Constant  Value=epsilon_w
  Gain : Gain  Gain=omega_w
  Gain1 : Gain  Gain=k_w
  Gain2 : Gain  Gain=A_w
  Gain5 : Gain  Gain=A_w*k_w
  Sum : Sum  Inputs=++-
  Trigonometric Function1 : Trigonometry  Operator=sincos
  Trigonometric Function2 : Trigonometry  Operator=atan
  direction : Gain  Gain=w_dir
  zeta(x,t) : Outport
  theta : Outport  Port=2
  wires:
  Sum/1 -> Trigonometric Function1/1
  direction/1 -> Gain/1
  x/1 -> Gain1/1
  Trigonometric Function1/1 -> Gain2/1
  Gain1/1 -> Sum/3
  t/1 -> direction/1
  Constant/1 -> Sum/1
  Gain2/1 -> zeta(x,t)/1  "zeta(x,t)"
  Gain/1 -> Sum/2
  Trigonometric Function1/2 -> Gain5/1
  Gain5/1 -> Trigonometric Function2/1
  Trigonometric Function2/1 -> theta/1

== system Simulator_3D/Subsystem2/Subsystem11/Subsystem1 ==
  note: Aw.Sin
  t : Inport
  x : Inport  Port=2
  Constant : Constant  Value=epsilon_w2
  Gain : Gain  Gain=omega_w2
  Gain1 : Gain  Gain=k_w2
  Gain2 : Gain  Gain=A_w2
  Gain5 : Gain  Gain=A_w2*k_w2
  Sum : Sum  Inputs=++-
  Trigonometric Function : Trigonometry  Operator=sincos
  Trigonometric Function1 : Trigonometry  Operator=atan
  direction : Gain  Gain=w_dir2
  zeta(x,t) : Outport
  theta : Outport  Port=2
  wires:
  Gain/1 -> Sum/2
  Gain2/1 -> zeta(x,t)/1  "zeta(x,t)"
  Constant/1 -> Sum/1
  t/1 -> direction/1
  Gain1/1 -> Sum/3
  Trigonometric Function/1 -> Gain2/1
  x/1 -> Gain1/1
  direction/1 -> Gain/1
  Sum/1 -> Trigonometric Function/1
  Gain5/1 -> Trigonometric Function1/1
  Trigonometric Function1/1 -> theta/1
  Trigonometric Function/2 -> Gain5/1

== system Simulator_3D/Subsystem2/Subsystem12/Subsystem ==
  note: Aw.Sin
  t : Inport
  x : Inport  Port=2
  Constant : Constant  Value=epsilon_w
  Gain : Gain  Gain=omega_w
  Gain1 : Gain  Gain=k_w
  Gain2 : Gain  Gain=A_w
  Gain5 : Gain  Gain=A_w*k_w
  Sum : Sum  Inputs=++-
  Trigonometric Function1 : Trigonometry  Operator=sincos
  Trigonometric Function2 : Trigonometry  Operator=atan
  direction : Gain  Gain=w_dir
  zeta(x,t) : Outport
  theta : Outport  Port=2
  wires:
  Trigonometric Function2/1 -> theta/1
  Gain5/1 -> Trigonometric Function2/1
  Trigonometric Function1/2 -> Gain5/1
  Gain/1 -> Sum/2
  Gain2/1 -> zeta(x,t)/1  "zeta(x,t)"
  Constant/1 -> Sum/1
  t/1 -> direction/1
  Gain1/1 -> Sum/3
  Trigonometric Function1/1 -> Gain2/1
  x/1 -> Gain1/1
  direction/1 -> Gain/1
  Sum/1 -> Trigonometric Function1/1

== system Simulator_3D/Subsystem2/Subsystem12/Subsystem1 ==
  note: Aw.Sin
  t : Inport
  x : Inport  Port=2
  Constant : Constant  Value=epsilon_w2
  Gain : Gain  Gain=omega_w2
  Gain1 : Gain  Gain=k_w2
  Gain2 : Gain  Gain=A_w2
  Gain5 : Gain  Gain=A_w2*k_w2
  Sum : Sum  Inputs=++-
  Trigonometric Function : Trigonometry  Operator=sincos
  Trigonometric Function1 : Trigonometry  Operator=atan
  direction : Gain  Gain=w_dir2
  zeta(x,t) : Outport
  theta : Outport  Port=2
  wires:
  Trigonometric Function/2 -> Gain5/1
  Trigonometric Function1/1 -> theta/1
  Gain5/1 -> Trigonometric Function1/1
  Sum/1 -> Trigonometric Function/1
  direction/1 -> Gain/1
  x/1 -> Gain1/1
  Trigonometric Function/1 -> Gain2/1
  Gain1/1 -> Sum/3
  t/1 -> direction/1
  Constant/1 -> Sum/1
  Gain2/1 -> zeta(x,t)/1  "zeta(x,t)"
  Gain/1 -> Sum/2

== system Simulator_3D/Subsystem2/Subsystem13/Subsystem ==
  note: Aw.Sin
  t : Inport
  x : Inport  Port=2
  Constant : Constant  Value=epsilon_w
  Gain : Gain  Gain=omega_w
  Gain1 : Gain  Gain=k_w
  Gain2 : Gain  Gain=A_w
  Gain5 : Gain  Gain=A_w*k_w
  Sum : Sum  Inputs=++-
  Trigonometric Function1 : Trigonometry  Operator=sincos
  Trigonometric Function2 : Trigonometry  Operator=atan
  direction : Gain  Gain=w_dir
  zeta(x,t) : Outport
  theta : Outport  Port=2
  wires:
  Sum/1 -> Trigonometric Function1/1
  direction/1 -> Gain/1
  x/1 -> Gain1/1
  Trigonometric Function1/1 -> Gain2/1
  Gain1/1 -> Sum/3
  t/1 -> direction/1
  Constant/1 -> Sum/1
  Gain2/1 -> zeta(x,t)/1  "zeta(x,t)"
  Gain/1 -> Sum/2
  Trigonometric Function1/2 -> Gain5/1
  Gain5/1 -> Trigonometric Function2/1
  Trigonometric Function2/1 -> theta/1

== system Simulator_3D/Subsystem2/Subsystem13/Subsystem1 ==
  note: Aw.Sin
  t : Inport
  x : Inport  Port=2
  Constant : Constant  Value=epsilon_w2
  Gain : Gain  Gain=omega_w2
  Gain1 : Gain  Gain=k_w2
  Gain2 : Gain  Gain=A_w2
  Gain5 : Gain  Gain=A_w2*k_w2
  Sum : Sum  Inputs=++-
  Trigonometric Function : Trigonometry  Operator=sincos
  Trigonometric Function1 : Trigonometry  Operator=atan
  direction : Gain  Gain=w_dir2
  zeta(x,t) : Outport
  theta : Outport  Port=2
  wires:
  Gain/1 -> Sum/2
  Gain2/1 -> zeta(x,t)/1  "zeta(x,t)"
  Constant/1 -> Sum/1
  t/1 -> direction/1
  Gain1/1 -> Sum/3
  Trigonometric Function/1 -> Gain2/1
  x/1 -> Gain1/1
  direction/1 -> Gain/1
  Sum/1 -> Trigonometric Function/1
  Gain5/1 -> Trigonometric Function1/1
  Trigonometric Function1/1 -> theta/1
  Trigonometric Function/2 -> Gain5/1

== system Simulator_3D/Subsystem2/Subsystem14/Subsystem ==
  note: Aw.Sin
  t : Inport
  x : Inport  Port=2
  Constant : Constant  Value=epsilon_w
  Gain : Gain  Gain=omega_w
  Gain1 : Gain  Gain=k_w
  Gain2 : Gain  Gain=A_w
  Gain5 : Gain  Gain=A_w*k_w
  Sum : Sum  Inputs=++-
  Trigonometric Function1 : Trigonometry  Operator=sincos
  Trigonometric Function2 : Trigonometry  Operator=atan
  direction : Gain  Gain=w_dir
  zeta(x,t) : Outport
  theta : Outport  Port=2
  wires:
  Trigonometric Function2/1 -> theta/1
  Gain5/1 -> Trigonometric Function2/1
  Trigonometric Function1/2 -> Gain5/1
  Gain/1 -> Sum/2
  Gain2/1 -> zeta(x,t)/1  "zeta(x,t)"
  Constant/1 -> Sum/1
  t/1 -> direction/1
  Gain1/1 -> Sum/3
  Trigonometric Function1/1 -> Gain2/1
  x/1 -> Gain1/1
  direction/1 -> Gain/1
  Sum/1 -> Trigonometric Function1/1

== system Simulator_3D/Subsystem2/Subsystem14/Subsystem1 ==
  note: Aw.Sin
  t : Inport
  x : Inport  Port=2
  Constant : Constant  Value=epsilon_w2
  Gain : Gain  Gain=omega_w2
  Gain1 : Gain  Gain=k_w2
  Gain2 : Gain  Gain=A_w2
  Gain5 : Gain  Gain=A_w2*k_w2
  Sum : Sum  Inputs=++-
  Trigonometric Function : Trigonometry  Operator=sincos
  Trigonometric Function1 : Trigonometry  Operator=atan
  direction : Gain  Gain=w_dir2
  zeta(x,t) : Outport
  theta : Outport  Port=2
  wires:
  Trigonometric Function/2 -> Gain5/1
  Trigonometric Function1/1 -> theta/1
  Gain5/1 -> Trigonometric Function1/1
  Sum/1 -> Trigonometric Function/1
  direction/1 -> Gain/1
  x/1 -> Gain1/1
  Trigonometric Function/1 -> Gain2/1
  Gain1/1 -> Sum/3
  t/1 -> direction/1
  Constant/1 -> Sum/1
  Gain2/1 -> zeta(x,t)/1  "zeta(x,t)"
  Gain/1 -> Sum/2

== system Simulator_3D/Subsystem2/Subsystem15/Subsystem ==
  note: Aw.Sin
  t : Inport
  x : Inport  Port=2
  Constant : Constant  Value=epsilon_w
  Gain : Gain  Gain=omega_w
  Gain1 : Gain  Gain=k_w
  Gain2 : Gain  Gain=A_w
  Gain5 : Gain  Gain=A_w*k_w
  Sum : Sum  Inputs=++-
  Trigonometric Function1 : Trigonometry  Operator=sincos
  Trigonometric Function2 : Trigonometry  Operator=atan
  direction : Gain  Gain=w_dir
  zeta(x,t) : Outport
  theta : Outport  Port=2
  wires:
  Sum/1 -> Trigonometric Function1/1
  direction/1 -> Gain/1
  x/1 -> Gain1/1
  Trigonometric Function1/1 -> Gain2/1
  Gain1/1 -> Sum/3
  t/1 -> direction/1
  Constant/1 -> Sum/1
  Gain2/1 -> zeta(x,t)/1  "zeta(x,t)"
  Gain/1 -> Sum/2
  Trigonometric Function1/2 -> Gain5/1
  Gain5/1 -> Trigonometric Function2/1
  Trigonometric Function2/1 -> theta/1

== system Simulator_3D/Subsystem2/Subsystem15/Subsystem1 ==
  note: Aw.Sin
  t : Inport
  x : Inport  Port=2
  Constant : Constant  Value=epsilon_w2
  Gain : Gain  Gain=omega_w2
  Gain1 : Gain  Gain=k_w2
  Gain2 : Gain  Gain=A_w2
  Gain5 : Gain  Gain=A_w2*k_w2
  Sum : Sum  Inputs=++-
  Trigonometric Function : Trigonometry  Operator=sincos
  Trigonometric Function1 : Trigonometry  Operator=atan
  direction : Gain  Gain=w_dir2
  zeta(x,t) : Outport
  theta : Outport  Port=2
  wires:
  Gain/1 -> Sum/2
  Gain2/1 -> zeta(x,t)/1  "zeta(x,t)"
  Constant/1 -> Sum/1
  t/1 -> direction/1
  Gain1/1 -> Sum/3
  Trigonometric Function/1 -> Gain2/1
  x/1 -> Gain1/1
  direction/1 -> Gain/1
  Sum/1 -> Trigonometric Function/1
  Gain5/1 -> Trigonometric Function1/1
  Trigonometric Function1/1 -> theta/1
  Trigonometric Function/2 -> Gain5/1

== system Simulator_3D/Subsystem2/Subsystem16/Subsystem ==
  note: Aw.Sin
  t : Inport
  x : Inport  Port=2
  Constant : Constant  Value=epsilon_w
  Gain : Gain  Gain=omega_w
  Gain1 : Gain  Gain=k_w
  Gain2 : Gain  Gain=A_w
  Gain5 : Gain  Gain=A_w*k_w
  Sum : Sum  Inputs=++-
  Trigonometric Function1 : Trigonometry  Operator=sincos
  Trigonometric Function2 : Trigonometry  Operator=atan
  direction : Gain  Gain=w_dir
  zeta(x,t) : Outport
  theta : Outport  Port=2
  wires:
  Trigonometric Function2/1 -> theta/1
  Gain5/1 -> Trigonometric Function2/1
  Trigonometric Function1/2 -> Gain5/1
  Gain/1 -> Sum/2
  Gain2/1 -> zeta(x,t)/1  "zeta(x,t)"
  Constant/1 -> Sum/1
  t/1 -> direction/1
  Gain1/1 -> Sum/3
  Trigonometric Function1/1 -> Gain2/1
  x/1 -> Gain1/1
  direction/1 -> Gain/1
  Sum/1 -> Trigonometric Function1/1

== system Simulator_3D/Subsystem2/Subsystem16/Subsystem1 ==
  note: Aw.Sin
  t : Inport
  x : Inport  Port=2
  Constant : Constant  Value=epsilon_w2
  Gain : Gain  Gain=omega_w2
  Gain1 : Gain  Gain=k_w2
  Gain2 : Gain  Gain=A_w2
  Gain5 : Gain  Gain=A_w2*k_w2
  Sum : Sum  Inputs=++-
  Trigonometric Function : Trigonometry  Operator=sincos
  Trigonometric Function1 : Trigonometry  Operator=atan
  direction : Gain  Gain=w_dir2
  zeta(x,t) : Outport
  theta : Outport  Port=2
  wires:
  Trigonometric Function/2 -> Gain5/1
  Trigonometric Function1/1 -> theta/1
  Gain5/1 -> Trigonometric Function1/1
  Sum/1 -> Trigonometric Function/1
  direction/1 -> Gain/1
  x/1 -> Gain1/1
  Trigonometric Function/1 -> Gain2/1
  Gain1/1 -> Sum/3
  t/1 -> direction/1
  Constant/1 -> Sum/1
  Gain2/1 -> zeta(x,t)/1  "zeta(x,t)"
  Gain/1 -> Sum/2

== system Simulator_3D/Subsystem2/Subsystem2/Subsystem ==
  note: Aw.Sin
  t : Inport
  x : Inport  Port=2
  Constant : Constant  Value=epsilon_w
  Gain : Gain  Gain=omega_w
  Gain1 : Gain  Gain=k_w
  Gain2 : Gain  Gain=A_w
  Gain5 : Gain  Gain=A_w*k_w
  Sum : Sum  Inputs=++-
  Trigonometric Function1 : Trigonometry  Operator=sincos
  Trigonometric Function2 : Trigonometry  Operator=atan
  direction : Gain  Gain=w_dir
  zeta(x,t) : Outport
  theta : Outport  Port=2
  wires:
  Sum/1 -> Trigonometric Function1/1
  direction/1 -> Gain/1
  x/1 -> Gain1/1
  Trigonometric Function1/1 -> Gain2/1
  Gain1/1 -> Sum/3
  t/1 -> direction/1
  Constant/1 -> Sum/1
  Gain2/1 -> zeta(x,t)/1  "zeta(x,t)"
  Gain/1 -> Sum/2
  Trigonometric Function1/2 -> Gain5/1
  Gain5/1 -> Trigonometric Function2/1
  Trigonometric Function2/1 -> theta/1

== system Simulator_3D/Subsystem2/Subsystem2/Subsystem1 ==
  note: Aw.Sin
  t : Inport
  x : Inport  Port=2
  Constant : Constant  Value=epsilon_w2
  Gain : Gain  Gain=omega_w2
  Gain1 : Gain  Gain=k_w2
  Gain2 : Gain  Gain=A_w2
  Gain5 : Gain  Gain=A_w2*k_w2
  Sum : Sum  Inputs=++-
  Trigonometric Function : Trigonometry  Operator=sincos
  Trigonometric Function1 : Trigonometry  Operator=atan
  direction : Gain  Gain=w_dir2
  zeta(x,t) : Outport
  theta : Outport  Port=2
  wires:
  Gain/1 -> Sum/2
  Gain2/1 -> zeta(x,t)/1  "zeta(x,t)"
  Constant/1 -> Sum/1
  t/1 -> direction/1
  Gain1/1 -> Sum/3
  Trigonometric Function/1 -> Gain2/1
  x/1 -> Gain1/1
  direction/1 -> Gain/1
  Sum/1 -> Trigonometric Function/1
  Gain5/1 -> Trigonometric Function1/1
  Trigonometric Function1/1 -> theta/1
  Trigonometric Function/2 -> Gain5/1

== system Simulator_3D/Subsystem2/Subsystem3/Subsystem ==
  note: Aw.Sin
  t : Inport
  x : Inport  Port=2
  Constant : Constant  Value=epsilon_w
  Gain : Gain  Gain=omega_w
  Gain1 : Gain  Gain=k_w
  Gain2 : Gain  Gain=A_w
  Gain5 : Gain  Gain=A_w*k_w
  Sum : Sum  Inputs=++-
  Trigonometric Function1 : Trigonometry  Operator=sincos
  Trigonometric Function2 : Trigonometry  Operator=atan
  direction : Gain  Gain=w_dir
  zeta(x,t) : Outport
  theta : Outport  Port=2
  wires:
  Sum/1 -> Trigonometric Function1/1
  direction/1 -> Gain/1
  x/1 -> Gain1/1
  Trigonometric Function1/1 -> Gain2/1
  Gain1/1 -> Sum/3
  t/1 -> direction/1
  Constant/1 -> Sum/1
  Gain2/1 -> zeta(x,t)/1  "zeta(x,t)"
  Gain/1 -> Sum/2
  Trigonometric Function1/2 -> Gain5/1
  Gain5/1 -> Trigonometric Function2/1
  Trigonometric Function2/1 -> theta/1

== system Simulator_3D/Subsystem2/Subsystem3/Subsystem1 ==
  note: Aw.Sin
  t : Inport
  x : Inport  Port=2
  Constant : Constant  Value=epsilon_w2
  Gain : Gain  Gain=omega_w2
  Gain1 : Gain  Gain=k_w2
  Gain2 : Gain  Gain=A_w2
  Gain5 : Gain  Gain=A_w2*k_w2
  Sum : Sum  Inputs=++-
  Trigonometric Function : Trigonometry  Operator=sincos
  Trigonometric Function1 : Trigonometry  Operator=atan
  direction : Gain  Gain=w_dir2
  zeta(x,t) : Outport
  theta : Outport  Port=2
  wires:
  Gain/1 -> Sum/2
  Gain2/1 -> zeta(x,t)/1  "zeta(x,t)"
  Constant/1 -> Sum/1
  t/1 -> direction/1
  Gain1/1 -> Sum/3
  Trigonometric Function/1 -> Gain2/1
  x/1 -> Gain1/1
  direction/1 -> Gain/1
  Sum/1 -> Trigonometric Function/1
  Gain5/1 -> Trigonometric Function1/1
  Trigonometric Function1/1 -> theta/1
  Trigonometric Function/2 -> Gain5/1

== system Simulator_3D/Subsystem2/Subsystem4/Subsystem ==
  note: Aw.Sin
  t : Inport
  x : Inport  Port=2
  Constant : Constant  Value=epsilon_w
  Gain : Gain  Gain=omega_w
  Gain1 : Gain  Gain=k_w
  Gain2 : Gain  Gain=A_w
  Gain5 : Gain  Gain=A_w*k_w
  Sum : Sum  Inputs=++-
  Trigonometric Function1 : Trigonometry  Operator=sincos
  Trigonometric Function2 : Trigonometry  Operator=atan
  direction : Gain  Gain=w_dir
  zeta(x,t) : Outport
  theta : Outport  Port=2
  wires:
  Trigonometric Function2/1 -> theta/1
  Gain5/1 -> Trigonometric Function2/1
  Trigonometric Function1/2 -> Gain5/1
  Gain/1 -> Sum/2
  Gain2/1 -> zeta(x,t)/1  "zeta(x,t)"
  Constant/1 -> Sum/1
  t/1 -> direction/1
  Gain1/1 -> Sum/3
  Trigonometric Function1/1 -> Gain2/1
  x/1 -> Gain1/1
  direction/1 -> Gain/1
  Sum/1 -> Trigonometric Function1/1

== system Simulator_3D/Subsystem2/Subsystem4/Subsystem1 ==
  note: Aw.Sin
  t : Inport
  x : Inport  Port=2
  Constant : Constant  Value=epsilon_w2
  Gain : Gain  Gain=omega_w2
  Gain1 : Gain  Gain=k_w2
  Gain2 : Gain  Gain=A_w2
  Gain5 : Gain  Gain=A_w2*k_w2
  Sum : Sum  Inputs=++-
  Trigonometric Function : Trigonometry  Operator=sincos
  Trigonometric Function1 : Trigonometry  Operator=atan
  direction : Gain  Gain=w_dir2
  zeta(x,t) : Outport
  theta : Outport  Port=2
  wires:
  Trigonometric Function/2 -> Gain5/1
  Trigonometric Function1/1 -> theta/1
  Gain5/1 -> Trigonometric Function1/1
  Sum/1 -> Trigonometric Function/1
  direction/1 -> Gain/1
  x/1 -> Gain1/1
  Trigonometric Function/1 -> Gain2/1
  Gain1/1 -> Sum/3
  t/1 -> direction/1
  Constant/1 -> Sum/1
  Gain2/1 -> zeta(x,t)/1  "zeta(x,t)"
  Gain/1 -> Sum/2

== system Simulator_3D/Subsystem2/Subsystem5/Subsystem ==
  note: Aw.Sin
  t : Inport
  x : Inport  Port=2
  Constant : Constant  Value=epsilon_w
  Gain : Gain  Gain=omega_w
  Gain1 : Gain  Gain=k_w
  Gain2 : Gain  Gain=A_w
  Gain5 : Gain  Gain=A_w*k_w
  Sum : Sum  Inputs=++-
  Trigonometric Function1 : Trigonometry  Operator=sincos
  Trigonometric Function2 : Trigonometry  Operator=atan
  direction : Gain  Gain=w_dir
  zeta(x,t) : Outport
  theta : Outport  Port=2
  wires:
  Sum/1 -> Trigonometric Function1/1
  direction/1 -> Gain/1
  x/1 -> Gain1/1
  Trigonometric Function1/1 -> Gain2/1
  Gain1/1 -> Sum/3
  t/1 -> direction/1
  Constant/1 -> Sum/1
  Gain2/1 -> zeta(x,t)/1  "zeta(x,t)"
  Gain/1 -> Sum/2
  Trigonometric Function1/2 -> Gain5/1
  Gain5/1 -> Trigonometric Function2/1
  Trigonometric Function2/1 -> theta/1

== system Simulator_3D/Subsystem2/Subsystem5/Subsystem1 ==
  note: Aw.Sin
  t : Inport
  x : Inport  Port=2
  Constant : Constant  Value=epsilon_w2
  Gain : Gain  Gain=omega_w2
  Gain1 : Gain  Gain=k_w2
  Gain2 : Gain  Gain=A_w2
  Gain5 : Gain  Gain=A_w2*k_w2
  Sum : Sum  Inputs=++-
  Trigonometric Function : Trigonometry  Operator=sincos
  Trigonometric Function1 : Trigonometry  Operator=atan
  direction : Gain  Gain=w_dir2
  zeta(x,t) : Outport
  theta : Outport  Port=2
  wires:
  Gain/1 -> Sum/2
  Gain2/1 -> zeta(x,t)/1  "zeta(x,t)"
  Constant/1 -> Sum/1
  t/1 -> direction/1
  Gain1/1 -> Sum/3
  Trigonometric Function/1 -> Gain2/1
  x/1 -> Gain1/1
  direction/1 -> Gain/1
  Sum/1 -> Trigonometric Function/1
  Gain5/1 -> Trigonometric Function1/1
  Trigonometric Function1/1 -> theta/1
  Trigonometric Function/2 -> Gain5/1

== system Simulator_3D/Subsystem2/Subsystem6/Subsystem ==
  note: Aw.Sin
  t : Inport
  x : Inport  Port=2
  Constant : Constant  Value=epsilon_w
  Gain : Gain  Gain=omega_w
  Gain1 : Gain  Gain=k_w
  Gain2 : Gain  Gain=A_w
  Gain5 : Gain  Gain=A_w*k_w
  Sum : Sum  Inputs=++-
  Trigonometric Function1 : Trigonometry  Operator=sincos
  Trigonometric Function2 : Trigonometry  Operator=atan
  direction : Gain  Gain=w_dir
  zeta(x,t) : Outport
  theta : Outport  Port=2
  wires:
  Trigonometric Function2/1 -> theta/1
  Gain5/1 -> Trigonometric Function2/1
  Trigonometric Function1/2 -> Gain5/1
  Gain/1 -> Sum/2
  Gain2/1 -> zeta(x,t)/1  "zeta(x,t)"
  Constant/1 -> Sum/1
  t/1 -> direction/1
  Gain1/1 -> Sum/3
  Trigonometric Function1/1 -> Gain2/1
  x/1 -> Gain1/1
  direction/1 -> Gain/1
  Sum/1 -> Trigonometric Function1/1

== system Simulator_3D/Subsystem2/Subsystem6/Subsystem1 ==
  note: Aw.Sin
  t : Inport
  x : Inport  Port=2
  Constant : Constant  Value=epsilon_w2
  Gain : Gain  Gain=omega_w2
  Gain1 : Gain  Gain=k_w2
  Gain2 : Gain  Gain=A_w2
  Gain5 : Gain  Gain=A_w2*k_w2
  Sum : Sum  Inputs=++-
  Trigonometric Function : Trigonometry  Operator=sincos
  Trigonometric Function1 : Trigonometry  Operator=atan
  direction : Gain  Gain=w_dir2
  zeta(x,t) : Outport
  theta : Outport  Port=2
  wires:
  Trigonometric Function/2 -> Gain5/1
  Trigonometric Function1/1 -> theta/1
  Gain5/1 -> Trigonometric Function1/1
  Sum/1 -> Trigonometric Function/1
  direction/1 -> Gain/1
  x/1 -> Gain1/1
  Trigonometric Function/1 -> Gain2/1
  Gain1/1 -> Sum/3
  t/1 -> direction/1
  Constant/1 -> Sum/1
  Gain2/1 -> zeta(x,t)/1  "zeta(x,t)"
  Gain/1 -> Sum/2
